simulink library "swblockset"  (R2015a)
settings: Solver=ode45  StartTime=0.0  StopTime=10.0  RelTol=1e-3
settings Model: Creator=Francescodario  LastModifiedBy=Francescodario

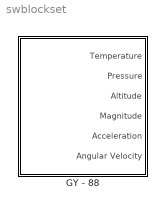
== system swblockset ==
  "GY - 88 " : Subsystem  mask(GY-88){S_T=0.02}
      mask prompts: S_T "Sample Time"
      mask help: This block will output data from GY-88 IMU

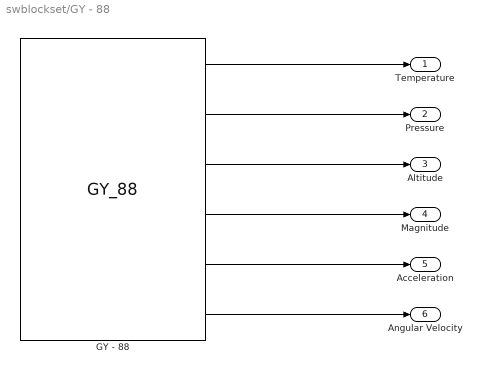
== system swblockset/GY - 88  ==
  "GY - 88 " : S-Function  InitFcn=try, set_param(gcb,'FunctionName','GY_88'), end  FunctionName=GY_88  Parameters=0.02  SFunctionModules=GY_88_wrapper  mask(S-Function Builder){}
      mask help: Simulink:masks:SFunctionBuilder_MD
      mask init:
      | val = [[.9  0.75 0.75 1 1 .9 .9 1]',[1 1 0.75 0.75 .9 .9 1 .9]'];try , sys = get_param(gcb,'SfunBuilderFcnName');if isempty(sys), sys = get_param(gcb,'FunctionName'); end,catch, sys = get_param(gcb,'FunctionName'); end
      settings: CopyFcn=set_param(gcbh,'LinkStatus','none')  PreSaveFcn=try, set_param(gcb,'FunctionName','GY_88'), end  OpenFcn=sfunctionwizard(gcbh)
      mask Display: plot(val(:,1),val(:,2)),disp(sys), port_label('output',1,'temperature'), port_label('output',2,'pressure'), port_label('output',3,'altitude'), port_label('output',4,'magnitude'), port_label('output',5,'acceleration'), port_label('output',6,'angular_velocity')
  Temperature : Outport
  Pressure : Outport  Port=2
  Altitude : Outport  Port=3
  Magnitude : Outport  Port=4
  Acceleration : Outport  Port=5
  Angular Velocity : Outport  Port=6
  wires:
  "GY - 88 "/5 -> Acceleration/1
  "GY - 88 "/3 -> Altitude/1
  "GY - 88 "/6 -> Angular Velocity/1
  "GY - 88 "/2 -> Pressure/1
  "GY - 88 "/4 -> Magnitude/1
  "GY - 88 "/1 -> Temperature/1
